simulink library "INT_CoAS_RlsCmpn"  (R2016b)
settings: Solver=VariableStepAuto  StartTime=0.0  StopTime=10.0  RelTol=1e-3
settings Model: Creator=Wollf  LastModifiedBy=Wollf

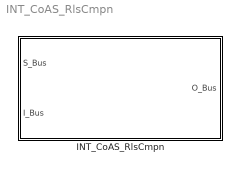
== system INT_CoAS_RlsCmpn ==
  INT_CoAS_RlsCmpn : Subsystem

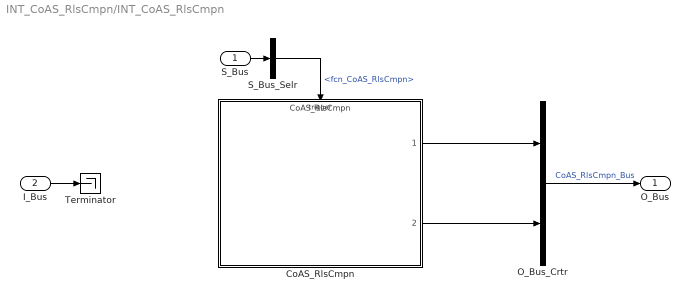
== system INT_CoAS_RlsCmpn/INT_CoAS_RlsCmpn ==
  S_Bus : Inport
  I_Bus : Inport  Port=2
  CoAS_RlsCmpn : ModelReference  ModelNameDialog=CoAS_RlsCmpn  SimulationMode=Normal  ModelReferenceVersion=1.5  TriggerPortName=function  TriggerPortTriggerType=function-call  TriggerPortStatesWhenEnabling=held
  O_Bus_Crtr : BusCreator  Inputs=2
  S_Bus_Selr : BusSelector  OutputSignals=fcn_CoAS_RlsCmpn
  Terminator : Terminator
  O_Bus : Outport
  wires:
  S_Bus_Selr/1 -> CoAS_RlsCmpn/Trigger  "<fcn_CoAS_RlsCmpn>"
  S_Bus/1 -> S_Bus_Selr/1
  I_Bus/1 -> Terminator/1
  O_Bus_Crtr/1 -> O_Bus/1  "CoAS_RlsCmpn_Bus"
  CoAS_RlsCmpn/1 -> O_Bus_Crtr/1
  CoAS_RlsCmpn/2 -> O_Bus_Crtr/2
